simulink model "program_simulink_2"  (R2024b)
settings: Solver=VariableStepAuto  StartTime=0.0  StopTime=2  MaxStep=0.001  RelTol=1e-3
undefined symbols (not defined in the file): L, R, Vs
libraries: simulink x1
settings Model: Creator=俞书阳  LastModifiedBy=user

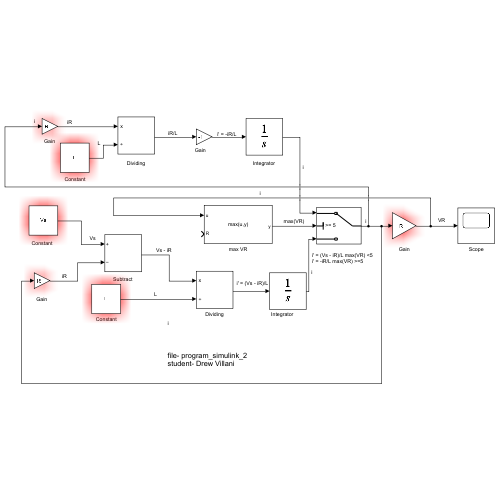
[thumbnail: Simulink's stored preview of the top-level diagram]
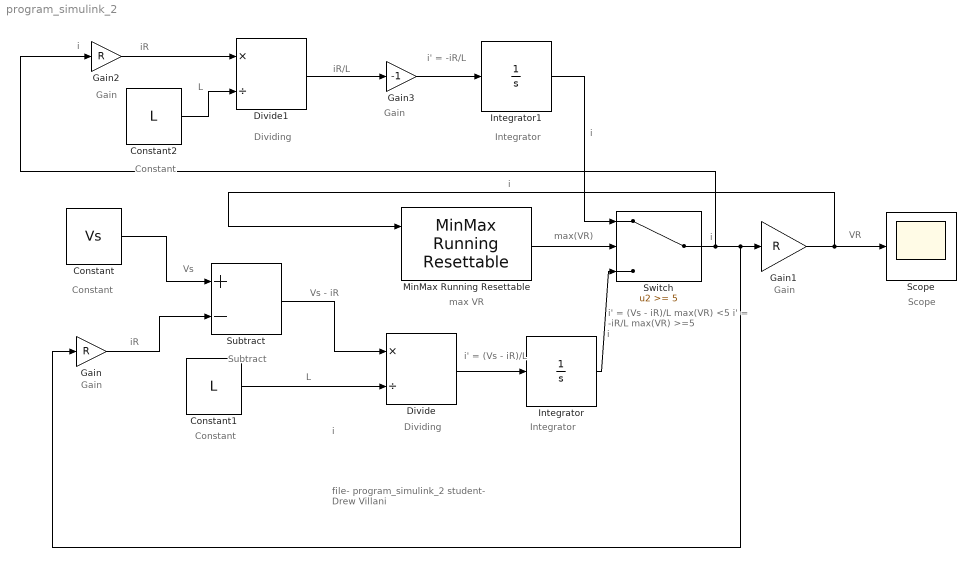
== system program_simulink_2 ==
  note: file- program_simulink_2
      | student- Drew Villani
  note: i' = (Vs - iR)/L max(VR) <5
      | i' = -iR/L max(VR) >=5
  note: i
  note: i' = -iR/L
  note: iR/L
  note: L
  note: i
  note: i' = (Vs - iR)/L
  note: Vs - iR
  note: L
  note: iR
  note: i
  note: max(VR)
  note: i
  note: VR
  note: i
  note: max VR
  note: Scope
  note: Integrator
  note: Dividing
  note: Gain
  note: Subtract
  note: Vs
  note: Constant
  note: Constant
  note: Constant
  note: Gain
  note: Gain
  note: Gain
  note: Dividing
  note: Integrator
  note: i
  note: iR
  Constant : Constant  Value=Vs
  Constant1 : Constant  Value=L
  Constant2 : Constant  Value=L
  Divide : Product  Inputs=*/
  Divide1 : Product  Inputs=*/
  Gain : Gain  Gain=R
  Gain1 : Gain  Gain=R
  Gain2 : Gain  Gain=R
  Gain3 : Gain  Gain=-1
  Integrator : Integrator
  Integrator1 : Integrator
  MinMax Running Resettable : simulink/Math Operations/MinMax Running Resettable  Function=max  vinit=0.0
  Scope : Scope
  Subtract : Sum  Inputs=+-
  Switch : Switch  Threshold=5  SaturateOnIntegerOverflow=off  InputSameDT=off
  wires:
  MinMax Running Resettable/1 -> Switch/2
  Gain/1 -> Subtract/2
  Constant/1 -> Subtract/1
  Subtract/1 -> Divide/1
  Constant1/1 -> Divide/2
  Divide/1 -> Integrator/1
  Integrator/1 -> Switch/3
  Switch/1 -> Gain/1, Gain1/1, Gain2/1
  Gain2/1 -> Divide1/1
  Constant2/1 -> Divide1/2
  Divide1/1 -> Gain3/1
  Integrator1/1 -> Switch/1
  Gain3/1 -> Integrator1/1
  Gain1/1 -> MinMax Running Resettable/1, Scope/1
